simulink model "exp2test1step"  (R2018b)
settings: Solver=FixedStepAuto  StartTime=0.0  StopTime=tspan  FixedStep=0.0001  RelTol=1e-3
values from neighbouring files (symbols this model uses):
  A1 = [ 0 1; -k/m -c/m]    [Lab2_Matlab.m]
  B1 = [ 0; 1/m]    [Lab2_Matlab.m]
  C1 = [1 0; 0 1]    [Lab2_Matlab.m]
  D1 = [0; 0]    [Lab2_Matlab.m]
  q0 = [ 0; 0]    [Lab2_Matlab.m]
settings Model: Creator=Zoe  LastModifiedBy=Zoe

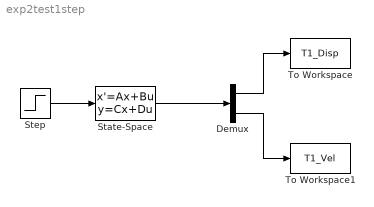
== system exp2test1step ==
  Demux : Demux  Outputs=2
  State-Space : StateSpace  A=A1  B=B1  C=C1  D=D1  InitialCondition=q0
  Step : Step  After=4  SampleTime=0
  To Workspace : ToWorkspace  VariableName=T1_Disp  SaveFormat=Timeseries  SampleTime=-1
  To Workspace1 : ToWorkspace  VariableName=T1_Vel  SaveFormat=Timeseries  SampleTime=-1
  wires:
  Step/1 -> State-Space/1
  State-Space/1 -> Demux/1
  Demux/1 -> To Workspace/1
  Demux/2 -> To Workspace1/1
